simulink model "DLC"  (R2022b)
settings: Solver=VariableStepAuto  StartTime=0.0  StopTime=10  RelTol=1e-3
libraries: commchan3 x2, simulink x2
settings Model: Creator=Suresh  LastModifiedBy=Suresh

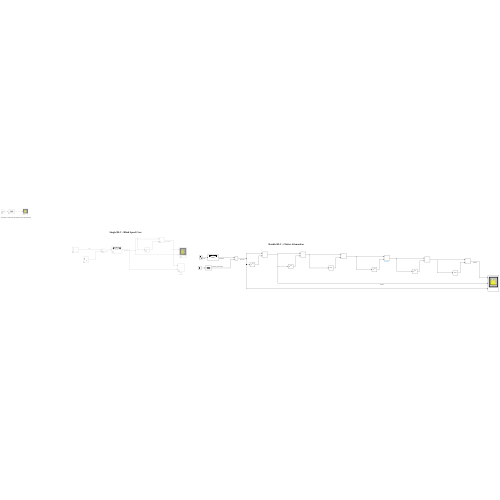
[thumbnail: Simulink's stored preview of the top-level diagram]
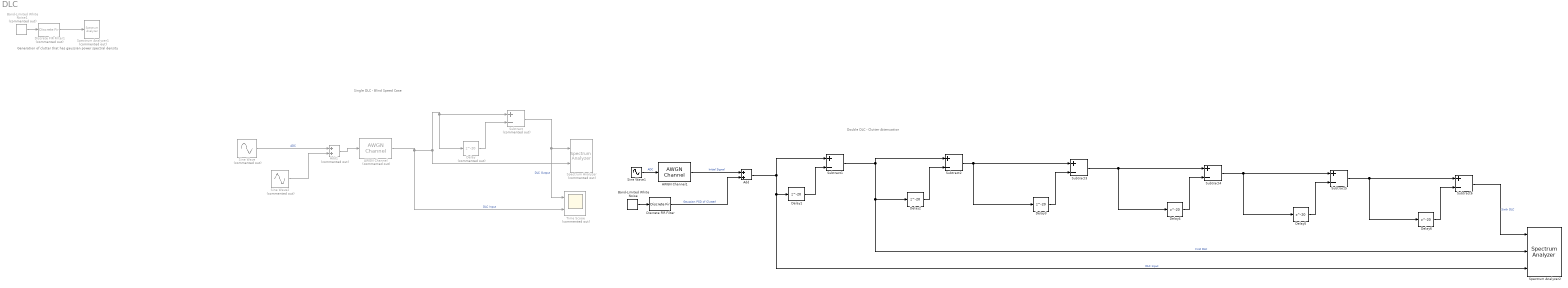
== system DLC ==
  note: Generation of clutter that has gaussian power spectral density
  note: Single DLC - Blind Speed Case
  note: Double DLC - Clutter Attenuation
  AWGN Channel : commchan3/AWGN Channel  Commented=on  InputProcessing=Columns as channels (frame based)  seed=67  noiseMode="Signal to noise ratio  (SNR)"  EbNodB=10  EsNodB=10  SNRdB=30  bitsPerSym=1  Ps=10  Tsym=1  variance=1
  AWGN Channel1 : commchan3/AWGN Channel  InputProcessing=Columns as channels (frame based)  seed=67  noiseMode="Signal to noise ratio  (SNR)"  EbNodB=10  EsNodB=10  SNRdB=30  bitsPerSym=1  Ps=10  Tsym=1  variance=1
  Add : Sum
  Add1 : Sum  Commented=on
  Band-Limited White Noise : simulink/Sources/Band-Limited White Noise  Cov=[0.01]  Ts=50e-6  seed=[23341]
  Band-Limited White Noise1 : simulink/Sources/Band-Limited White Noise  Commented=on  Cov=[0.01]  Ts=50e-6  seed=[23341]
  Delay : Delay  Commented=on  DelayLength=20  SampleTime=50e-6
  Delay{1..6} (6 alike) : Delay  DelayLength=20  SampleTime=50e-6
  Discrete FIR Filter : DiscreteFir  Coefficients="[3.98420139652326e-06\t1.37878093532435e-05\t4.40418068449166e-05\t0.000129852662228866\t0.000353388538457777\t0.000887707590788669\t0.00205827443145017\t0.00440506677943770\t0.00870197008251853\t0.0158671361027577\t0.0267051720299709\t0.0414866229979718\t0.0594889990276258\t0.0787374072908141\t0.0961925483684035\t0.108471993725238\t0.112904093109483\t0.108471993725238\t0.0961925483684035\t0.0787374072908141\t0.0594889990276258\t0.0414866229979718\t0.0267051720299709\t0.0158671361027577\t0.00870197008251853\t0.00440506677943770\t0.00205827443145017\t0.000887707590788669\t0.000353388538457777\t0.000129852662228866\t4.40418068449166e-05\t1.37878093532435e-05\t3.98420139652326e-06]"  SampleTime=0.001
  Discrete FIR Filter1 : DiscreteFir  Commented=on  Coefficients="[3.98420139652326e-06\t1.37878093532435e-05\t4.40418068449166e-05\t0.000129852662228866\t0.000353388538457777\t0.000887707590788669\t0.00205827443145017\t0.00440506677943770\t0.00870197008251853\t0.0158671361027577\t0.0267051720299709\t0.0414866229979718\t0.0594889990276258\t0.0787374072908141\t0.0961925483684035\t0.108471993725238\t0.112904093109483\t0.108471993725238\t0.0961925483684035\t0.0787374072908141\t0.0594889990276258\t0.0414866229979718\t0.0267051720299709\t0.0158671361027577\t0.00870197008251853\t0.00440506677943770\t0.00205827443145017\t0.000887707590788669\t0.000353388538457777\t0.000129852662228866\t4.40418068449166e-05\t1.37878093532435e-05\t3.98420139652326e-06]"  SampleTime=0.001
  Sine Wave : Sin  Commented=on  Amplitude=2  Frequency=2*pi*2600  SampleTime=50e-6
  Sine Wave1 : Sin  Frequency=2*pi*2600  SampleTime=50e-6
  Sine Wave2 : Sin  Commented=on  Frequency=2*pi*2000  SampleTime=50e-6
  Spectrum Analyzer : SpectrumAnalyzer  Commented=on  NumInputPorts=2
  Spectrum Analyzer1 : SpectrumAnalyzer  Commented=on
  Spectrum Analyzer2 : SpectrumAnalyzer  NumInputPorts=3
  Subtract : Sum  Commented=on  Inputs=+-
  Subtract{1..6} (6 alike) : Sum  Inputs=+-
  Time Scope : Scope  Commented=on  NumInputPorts=2
  wires:
  Sine Wave/1 -> Add1/1  "ADC"
  Subtract/1 -> Time Scope/1, Spectrum Analyzer/1  "DLC Output"
  Delay/1 -> Subtract/2
  AWGN Channel/1 -> Time Scope/2, Spectrum Analyzer/2, Delay/1, Subtract/1  "DLC Input"
  AWGN Channel1/1 -> Add/1  "Initial Signal"
  Delay1/1 -> Subtract1/2
  Subtract1/1 -> Subtract2/1, Spectrum Analyzer2/2, Delay2/1  "First DLC"
  Delay2/1 -> Subtract2/2
  Sine Wave1/1 -> AWGN Channel1/1  "ADC"
  Add/1 -> Spectrum Analyzer2/3, Delay1/1, Subtract1/1  "DLC Input"
  Discrete FIR Filter/1 -> Add/2  "Gaussian PSD of Clutterl"
  Sine Wave2/1 -> Add1/2
  Add1/1 -> AWGN Channel/1
  Band-Limited White Noise/1 -> Discrete FIR Filter/1
  Discrete FIR Filter1/1 -> Spectrum Analyzer1/1
  Band-Limited White Noise1/1 -> Discrete FIR Filter1/1
  Delay3/1 -> Subtract3/2
  Subtract2/1 -> Delay3/1, Subtract3/1
  Delay4/1 -> Subtract4/2
  Subtract3/1 -> Delay4/1, Subtract4/1
  Delay5/1 -> Subtract5/2
  Subtract4/1 -> Delay5/1, Subtract5/1
  Delay6/1 -> Subtract6/2
  Subtract5/1 -> Delay6/1, Subtract6/1
  Subtract6/1 -> Spectrum Analyzer2/1  "Sixth DLC"
